simulink model "DCMotor"  (R2019a)
settings: Solver=ode23  StartTime=0.0  StopTime=5  RelTol=1e-3
libraries: powerlib x4, BELBICtoolbox x1
settings Model: Creator=pavan  LastModifiedBy=pavan

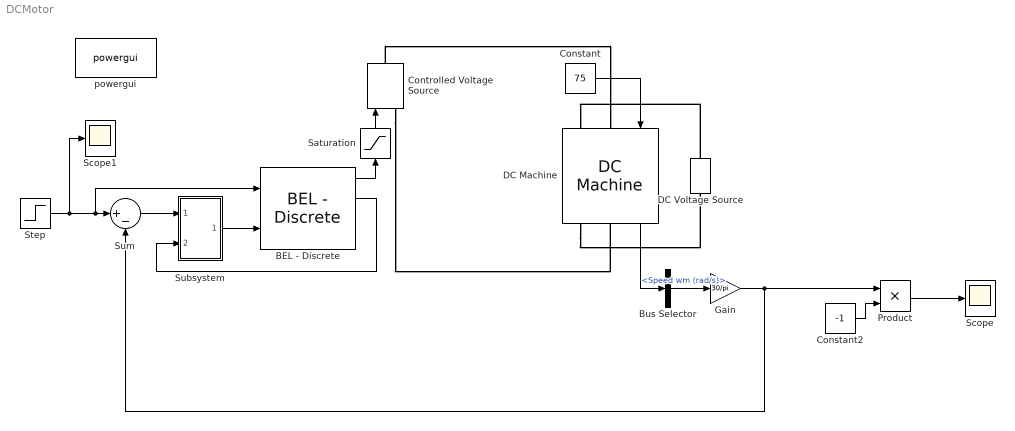
== system DCMotor ==
  BEL - Discrete : BELBICtoolbox/Discrete-time/BEL - Discrete  alfa=0.1  beta=0.01  V=30  Vth=25  W=0.001  T=5e-0
      settings: SourceProductName=BELBIC Toolbox
  Bus Selector : BusSelector  OutputSignals=Speed wm (rad/s)
  Constant : Constant  Value=75
  Constant2 : Constant  Value=-1
  Controlled Voltage Source : powerlib/Electrical Sources/Controlled Voltage Source  Initialize=on  Source_Type=DC  Amplitude=240  Phase=0  Frequency=50  Measurements=None
      settings: SourceProductName=Simscape Electrical
  DC Machine : powerlib/Machines/DC Machine  PresetModel=01: 5HP 240V 1750RPM Field:300V  MechanicalLoad=Torque TL  FieldType=Wound  ShowDetailedParameters=on  MeasurementBus=off  RLa=[2.581 0.028]  RLf=[281.3 156]  Laf=0.9483  MachineConstant=Torque constant (N.m/A)  Ke=1.8  Kt=1.8  J=0.02215  Bm=0.002953  Tf=0.5161  w0=1  Ifinit=1  TsPowergui=0  TsBlock=-1
      settings: SourceProductName=Simscape Electrical
  DC Voltage Source : powerlib/Electrical Sources/DC Voltage Source  Amplitude=300  Measurements=None
      settings: SourceProductName=Simscape Electrical
  Gain : Gain  Gain=30/pi
  Product : Product
  Saturation : Saturate  UpperLimit=1  LowerLimit=0
  Scope : Scope
  Scope1 : Scope
  Step : Step  After=1700  SampleTime=0
  Subsystem : Subsystem
  Sum : Sum  Inputs=|+-
  powergui : powerlib/powergui  Priority=1  SimulationMode=Discrete  SampleTime=50e-6  frequency=60  Iterations=50  frequencyindice=0  Pbase=100e6  ErrMax=1e-4  UnitsV=kV  UnitsW=MW  buscounter=0  FunctionMessages=off  echomessages=off  EnableUseOfTLC=off  CurrentSourceSwitches=off  DisableSnubberDevices=off  DisableRonSwitches=off  DisableVfSwitches=off  DisplayEquations=off  AutomaticDiscreteSolvers=off  SolverType=Tustin/Backward Euler (TBE)  Interpol=off  ExternalGateDelay=off  methode=off  Ts=100  x0status=blocks  SPID=on  SwTol=0  HookPort=off  NonlinearTolerance=0  nMaxIteration=15  ContinueOnMaxIteration=off  RestoreLinks=warning  ResistiveCurrentMeasurement=off  Frange=[0:2:500]  Ylog=off  Xlog=on  ShowGrid=off  save=off  variable=ZData  structure=0  ZoomFFT=off  StartTime=0.0  cycles=1  DisplayStyle=1  fundamental=60  FreqAxis=off  MaxFrequency=1000  frequencyindicesteady=1  RmsSteady=1  display=off
      settings: SourceProductName=Simscape Electrical
  wires:
  Bus Selector/1 -> Gain/1  "<Speed wm (rad/s)>"
  Step/1 -> Scope1/1, BEL - Discrete/1, Sum/1
  DC Machine/1 -> Bus Selector/1
  Subsystem/1(Out1) -> BEL - Discrete/2
  Sum/1 -> Subsystem/1(In1)
  Constant/1 -> DC Machine/1
  Product/1 -> Scope/1
  Constant2/1 -> Product/2
  Saturation/1 -> Controlled Voltage Source/1
  BEL - Discrete/1 -> Saturation/1
  Gain/1 -> Product/1, Sum/2
  BEL - Discrete/2 -> Subsystem/2(In2)
  connections:
  DC Voltage Source/RConn1 -- DC Machine/LConn2
  DC Machine/RConn2 -- DC Voltage Source/LConn1
  Controlled Voltage Source/RConn1 -- DC Machine/LConn1
  Controlled Voltage Source/LConn1 -- DC Machine/RConn1

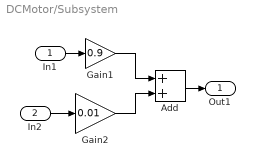
== system DCMotor/Subsystem ==
  In1 : Inport
  In2 : Inport  Port=2
  Add : Sum
  Gain1 : Gain  Gain=0.9
  Gain2 : Gain  Gain=0.01
  Out1 : Outport
  wires:
  In1/1 -> Gain1/1
  Gain2/1 -> Add/2
  In2/1 -> Gain2/1
  Add/1 -> Out1/1
  Gain1/1 -> Add/1
